simulink model "simulation"  (R2017b)
settings: Solver=VariableStepAuto  StartTime=0.0  StopTime=10.0  RelTol=1e-3
settings Model: Creator=Juan  LastModifiedBy=Juan

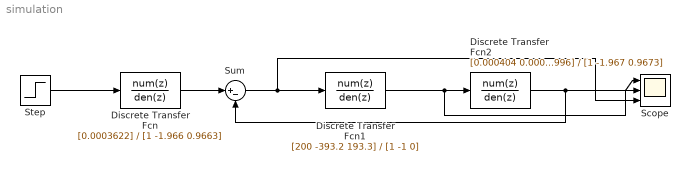
== system simulation ==
  Discrete Transfer Fcn : DiscreteTransferFcn  Numerator=[0.0003622]  Denominator=[1 -1.966 0.9663]  SampleTime=0.005
  Discrete Transfer Fcn1 : DiscreteTransferFcn  Numerator=[200 -393.2 193.3]  Denominator=[1 -1 0]  SampleTime=0.005
  Discrete Transfer Fcn2 : DiscreteTransferFcn  Numerator=[0.000404 0.0003996]  Denominator=[1 -1.967 0.9673]  SampleTime=0.005
  Scope : Scope  NumInputPorts=3
  Step : Step  SampleTime=0
  Sum : Sum  Inputs=|+-
  wires:
  Step/1 -> Discrete Transfer Fcn/1
  Discrete Transfer Fcn/1 -> Sum/1
  Discrete Transfer Fcn1/1 -> Scope/2, Discrete Transfer Fcn2/1
  Discrete Transfer Fcn2/1 -> Sum/2, Scope/1
  Sum/1 -> Scope/3, Discrete Transfer Fcn1/1
